simulink model "bh_compare_SM_vs_HAND_quad_and_spin_props"  (R2021b)
settings: Solver=ode23t  StartTime=0.0  StopTime=200  FixedStep=0.001  RelTol=1e-5  EnableMultiTasking=on
undefined symbols (not defined in the file or in its folder): P_elec, P_mot, P_one_prop, P_rot, P_veh, P_veh_no_props, sigbuilder_block, X, xme_dot_0, Y, Z
libraries: fl_lib x85, simulink_extras x40, nesl_utility x35, slpidlib x24, bh_6dof_LIBRARY x24, sm_lib x23, fl_ps_legacy_lib x7, simulink x2
(part 4 of 6)

== system bh_compare_SM_vs_HAND_quad_and_spin_props/CONT_SYS W_MOT_CMDS/MOTOR_sys/MOTOR_1 ==
  note: motor with PROPELLER
  w_CMD : Inport
  Bus Selector1 : BusSelector  OutputSignals=Elec.i,TQ_mot.Kt_i
  Lift : Scope  NumInputPorts=3
  MOTOR_PARAMS_STRUCT : bh_6dof_LIBRARY/MODELS/DC Motor_and_gearhead  K=P_mot.Ka  B=P_mot.b  J=P_mot.I  R=P_mot.R  L=P_mot.L  Kb=P_mot.Ke  ID=P_mot.ID
  Mux : Mux  Inputs=2
  PI_CONT : slpidlib/PID Controller  Controller=PI  Form=Parallel  TimeDomain=Continuous-time  UseExternalTs=off  SampleTime=-1  IntegratorMethod=Forward Euler  FilterMethod=Forward Euler  ControllerParametersSource=internal  P=2.97678216835849  I=24.9655384194189  D=-0.0417302954853434  UseFilter=on  N=6.67624174583517  TunerSelectOption=Transfer Function Based (PID Tuner App)  InitialConditionSource=internal  InitialConditionForIntegrator=0  InitialConditionForFilter=0  DifferentiatorICPrevScaledInput=0  ExternalReset=none  TrackingMode=off  Kt=1  LimitOutput=off  SatLimitsSource=internal  UpperSaturationLimit=inf  LowerSaturationLimit=-inf  LinearizeAsGain=on  AntiWindupMode=none  Kb=1  POutMin=[]  POutMax=[]  IOutMin=[]  IOutMax=[]  DOutMin=[]  DOutMax=[]  NOutMin=[]  NOutMax=[]  SumOutMin=[]  SumOutMax=[]  SaturationOutMin=[]  SaturationOutMax=[]  PParamMin=[]  PParamMax=[]  IParamMin=[]  IParamMax=[]  DParamMin=[]  DParamMax=[]  NParamMin=[]  NParamMax=[]  KbParamMin=[]  KbParamMax=[]  KtParamMin=[]  KtParamMax=[]  KbOutMin=[]  KbOutMax=[]  KtOutMin=[]  KtOutMax=[]  IntegratorOutMin=[]  IntegratorOutMax=[]  FilterOutMin=[]  FilterOutMax=[]  SumI1OutMin=[]  SumI1OutMax=[]  SumI2OutMin=[]  SumI2OutMax=[]  SumI3OutMin=[]  SumI3OutMax=[]  SumI4OutMin=[]  SumI4OutMax=[]  SumDOutMin=[]  SumDOutMax=[]  DifferentiatorOutMin=[]  DifferentiatorOutMax=[]  FilterDiffOutCoefMin=[]  FilterDiffOutCoefMax=[]  ReciprocalOutMin=[]  ReciprocalOutMax=[]  SumDenOutMin=[]  SumDenOutMax=[]  SumNumOutMin=[]  SumNumOutMax=[]  DivideOutMin=[]  DivideOutMax=[]  UdiffTsProdOutMin=[]  UdiffTsProdOutMax=[]  NTsProdOutMin=[]  NTsProdOutMax=[]  UintegralTsProdOutMin=[]  UintegralTsProdOutMax=[]  UngainTsProdOutMin=[]  UngainTsProdOutMax=[]  IntegratorContinuousStateAttributes=''  IntegratorStateMustResolveToSignalObject=off  IntegratorRTWStateStorageClass=Auto  FilterContinuousStateAttributes=''  FilterStateMustResolveToSignalObject=off  FilterRTWStateStorageClass=Auto  ParallelPVariant=InternalParameters  IdealPVariant=Disabled  IVariant=InternalParameters  DVariant=Disabled  IntegratorVariant=Continuous  SatVariant=Disabled  AWVariant=Passthrough  PCopyVariant=Disabled  TRVariant=Disabled  FdbkBlocksVariant=Forward  IdealPFdbkVariant=Disabled  SatFdbkVariant=Disabled  DerivativeFilterVariant=Disabled  NVariant=Disabled  NCopyVariant=Disabled_SignalSpec  FilterICVariant=Disabled  IntegratorICVariant=InternalICs  ExternalResetVariant=Disabled  TRSumVariant=Passthrough  SumFdbkVariant=Disabled  SumVariant=Sum_PI  TsampFilterVariant=InternalTs  TsampNgainVariant=Passthrough  TsampIntegralVariant=Passthrough  ExternalSaturationOutDataTypeStr=Inherit: Same as second input
  RPS_Lift_TG_drag : Scope  NumInputPorts=3
  Scope3 : Scope  NumInputPorts=4
  Sum1 : Sum  Inputs=|+-
  Terminator : Terminator
  VOLTAGE Saturation : Saturate  UpperLimit=P_elec.V_mot_max  LowerLimit=P_elec.V_mot_min
      settings: AttributesFormatString=|
      | Vmax = %<UpperLimit>
      | Vmin = %<LowerLimit>
  prefilter : Subsystem  mask(Derivative Estimation){wn=2*pi*5, p=1}
      mask prompts: wn "Natural frequency, wn (rad/sec)"; p "Damping ratio, p"
      mask help:
      | A simple derivative estimator using a 2nd order representation between input and output.
      |
      | The integrators use a discrete FORWARd Euler rule, and a sample time needs to be specified.
      mask init:
      | str1 = sprintf('wn = %.2f', wn);
      | str2 = sprintf('p  = %.2f', p);
      | %str3 = sprintf('dt = %.2f', dt);
      | %str = char(str1,str2,str3);
      | %str3 = sprintf('dt = %.2f', dt);
      | str = char(str1,str2);
      mask Display: disp(str)
  w_to_RPS : bh_6dof_LIBRARY/MODELS/w_to_RPS  SystemSampleTime=-1  VariantActivationTime=update diagram  Latency=0  AutoFrameSizeCalculation=off
  w_to_RPS1 : bh_6dof_LIBRARY/MODELS/w_to_RPS  SystemSampleTime=-1  VariantActivationTime=update diagram  Latency=0  AutoFrameSizeCalculation=off
  w_to_TQ_drag : bh_6dof_LIBRARY/MODELS/w_to_TQ_drag  k=P_one_prop.TWIST_per_w2
  w_to_Thrust : bh_6dof_LIBRARY/MODELS/w_to_Thrust  k=P_one_prop.LIFT_per_w2
  w : Outport  VectorParamsAs1DForOutWhenUnconnected=off
  wires:
  VOLTAGE Saturation/1 -> Lift/1, MOTOR_PARAMS_STRUCT/1  "VOLTS"
  [TQdrag] -> RPS_Lift_TG_drag/3  "TQdrag"
  Sum1/1 -> PI_CONT/1
  w_to_TQ_drag/1 -> [TQdrag], MOTOR_PARAMS_STRUCT/2, Scope3/4
  [LIFT] -> RPS_Lift_TG_drag/2  "LIFT"
  [wRPS_YES_prop] -> RPS_Lift_TG_drag/1  "RPS"
  w_to_Thrust/1 -> [LIFT]
  w_to_RPS/1 -> [wRPS_YES_prop], Scope3/1  "RPS"
  Bus Selector1/1 -> Scope3/2  "<i>"
  MOTOR_PARAMS_STRUCT/2 -> Bus Selector1/1
  Bus Selector1/2 -> Scope3/3  "<Kt_i>"
  MOTOR_PARAMS_STRUCT/1 -> w_to_RPS/1, [w], w/1, w_to_Thrust/1, w_to_TQ_drag/1
  [w] -> Sum1/2
  [LIFT] -> Lift/2  "LIFT"
  Mux/1 -> w_to_RPS1/1  "w"
  [w] -> Mux/2
  w_to_RPS1/1 -> Lift/3  "w_RPS"
  PI_CONT/1 -> VOLTAGE Saturation/1  "VOLTS"
  w_CMD/1 -> prefilter/1(U)  "w_rad_per_sec"
  prefilter/1(U_filt) -> Mux/1, Sum1/1
  prefilter/2(U_DOT) -> Terminator/1

== system bh_compare_SM_vs_HAND_quad_and_spin_props/CONT_SYS W_MOT_CMDS/MOTOR_sys/MOTOR_2 ==
  note: motor with PROPELLER
  w_CMD : Inport
  Bus Selector1 : BusSelector  OutputSignals=Elec.i,TQ_mot.Kt_i
  Lift : Scope  NumInputPorts=3
  MOTOR_PARAMS_STRUCT : bh_6dof_LIBRARY/MODELS/DC Motor_and_gearhead  K=P_mot.Ka  B=P_mot.b  J=P_mot.I  R=P_mot.R  L=P_mot.L  Kb=P_mot.Ke  ID=P_mot.ID
  Mux : Mux  Inputs=2
  PI_CONT : slpidlib/PID Controller  Controller=PI  Form=Parallel  TimeDomain=Continuous-time  UseExternalTs=off  SampleTime=-1  IntegratorMethod=Forward Euler  FilterMethod=Forward Euler  ControllerParametersSource=internal  P=2.97678216835849  I=24.9655384194189  D=-0.0417302954853434  UseFilter=on  N=6.67624174583517  TunerSelectOption=Transfer Function Based (PID Tuner App)  InitialConditionSource=internal  InitialConditionForIntegrator=0  InitialConditionForFilter=0  DifferentiatorICPrevScaledInput=0  ExternalReset=none  TrackingMode=off  Kt=1  LimitOutput=off  SatLimitsSource=internal  UpperSaturationLimit=inf  LowerSaturationLimit=-inf  LinearizeAsGain=on  AntiWindupMode=none  Kb=1  POutMin=[]  POutMax=[]  IOutMin=[]  IOutMax=[]  DOutMin=[]  DOutMax=[]  NOutMin=[]  NOutMax=[]  SumOutMin=[]  SumOutMax=[]  SaturationOutMin=[]  SaturationOutMax=[]  PParamMin=[]  PParamMax=[]  IParamMin=[]  IParamMax=[]  DParamMin=[]  DParamMax=[]  NParamMin=[]  NParamMax=[]  KbParamMin=[]  KbParamMax=[]  KtParamMin=[]  KtParamMax=[]  KbOutMin=[]  KbOutMax=[]  KtOutMin=[]  KtOutMax=[]  IntegratorOutMin=[]  IntegratorOutMax=[]  FilterOutMin=[]  FilterOutMax=[]  SumI1OutMin=[]  SumI1OutMax=[]  SumI2OutMin=[]  SumI2OutMax=[]  SumI3OutMin=[]  SumI3OutMax=[]  SumI4OutMin=[]  SumI4OutMax=[]  SumDOutMin=[]  SumDOutMax=[]  DifferentiatorOutMin=[]  DifferentiatorOutMax=[]  FilterDiffOutCoefMin=[]  FilterDiffOutCoefMax=[]  ReciprocalOutMin=[]  ReciprocalOutMax=[]  SumDenOutMin=[]  SumDenOutMax=[]  SumNumOutMin=[]  SumNumOutMax=[]  DivideOutMin=[]  DivideOutMax=[]  UdiffTsProdOutMin=[]  UdiffTsProdOutMax=[]  NTsProdOutMin=[]  NTsProdOutMax=[]  UintegralTsProdOutMin=[]  UintegralTsProdOutMax=[]  UngainTsProdOutMin=[]  UngainTsProdOutMax=[]  IntegratorContinuousStateAttributes=''  IntegratorStateMustResolveToSignalObject=off  IntegratorRTWStateStorageClass=Auto  FilterContinuousStateAttributes=''  FilterStateMustResolveToSignalObject=off  FilterRTWStateStorageClass=Auto  ParallelPVariant=InternalParameters  IdealPVariant=Disabled  IVariant=InternalParameters  DVariant=Disabled  IntegratorVariant=Continuous  SatVariant=Disabled  AWVariant=Passthrough  PCopyVariant=Disabled  TRVariant=Disabled  FdbkBlocksVariant=Forward  IdealPFdbkVariant=Disabled  SatFdbkVariant=Disabled  DerivativeFilterVariant=Disabled  NVariant=Disabled  NCopyVariant=Disabled_SignalSpec  FilterICVariant=Disabled  IntegratorICVariant=InternalICs  ExternalResetVariant=Disabled  TRSumVariant=Passthrough  SumFdbkVariant=Disabled  SumVariant=Sum_PI  TsampFilterVariant=InternalTs  TsampNgainVariant=Passthrough  TsampIntegralVariant=Passthrough  ExternalSaturationOutDataTypeStr=Inherit: Same as second input
  RPS_Lift_TG_drag : Scope  NumInputPorts=3
  Scope3 : Scope  NumInputPorts=4
  Sum1 : Sum  Inputs=|+-
  Terminator : Terminator
  VOLTAGE Saturation : Saturate  UpperLimit=P_elec.V_mot_max  LowerLimit=P_elec.V_mot_min
      settings: AttributesFormatString=|
      | Vmax = %<UpperLimit>
      | Vmin = %<LowerLimit>
  prefilter : Subsystem  mask(Derivative Estimation){wn=2*pi*5, p=1}
      mask prompts: wn "Natural frequency, wn (rad/sec)"; p "Damping ratio, p"
      mask help:
      | A simple derivative estimator using a 2nd order representation between input and output.
      |
      | The integrators use a discrete FORWARd Euler rule, and a sample time needs to be specified.
      mask init:
      | str1 = sprintf('wn = %.2f', wn);
      | str2 = sprintf('p  = %.2f', p);
      | %str3 = sprintf('dt = %.2f', dt);
      | %str = char(str1,str2,str3);
      | %str3 = sprintf('dt = %.2f', dt);
      | str = char(str1,str2);
      mask Display: disp(str)
  w_to_RPS : bh_6dof_LIBRARY/MODELS/w_to_RPS  SystemSampleTime=-1  VariantActivationTime=update diagram  Latency=0  AutoFrameSizeCalculation=off
  w_to_RPS1 : bh_6dof_LIBRARY/MODELS/w_to_RPS  SystemSampleTime=-1  VariantActivationTime=update diagram  Latency=0  AutoFrameSizeCalculation=off
  w_to_TQ_drag : bh_6dof_LIBRARY/MODELS/w_to_TQ_drag  k=P_one_prop.TWIST_per_w2
  w_to_Thrust : bh_6dof_LIBRARY/MODELS/w_to_Thrust  k=P_one_prop.LIFT_per_w2
  w : Outport  VectorParamsAs1DForOutWhenUnconnected=off
  wires:
  VOLTAGE Saturation/1 -> Lift/1, MOTOR_PARAMS_STRUCT/1  "VOLTS"
  [TQdrag] -> RPS_Lift_TG_drag/3  "TQdrag"
  Sum1/1 -> PI_CONT/1
  w_to_TQ_drag/1 -> [TQdrag], MOTOR_PARAMS_STRUCT/2, Scope3/4
  [LIFT] -> RPS_Lift_TG_drag/2  "LIFT"
  [wRPS_YES_prop] -> RPS_Lift_TG_drag/1  "RPS"
  w_to_Thrust/1 -> [LIFT]
  w_to_RPS/1 -> [wRPS_YES_prop], Scope3/1  "RPS"
  Bus Selector1/1 -> Scope3/2  "<i>"
  MOTOR_PARAMS_STRUCT/2 -> Bus Selector1/1
  Bus Selector1/2 -> Scope3/3  "<Kt_i>"
  MOTOR_PARAMS_STRUCT/1 -> w_to_RPS/1, [w], w/1, w_to_Thrust/1, w_to_TQ_drag/1
  [w] -> Sum1/2
  [LIFT] -> Lift/2  "LIFT"
  Mux/1 -> w_to_RPS1/1  "w"
  [w] -> Mux/2
  w_to_RPS1/1 -> Lift/3  "w_RPS"
  PI_CONT/1 -> VOLTAGE Saturation/1  "VOLTS"
  w_CMD/1 -> prefilter/1(U)  "w_rad_per_sec"
  prefilter/1(U_filt) -> Mux/1, Sum1/1
  prefilter/2(U_DOT) -> Terminator/1

== system bh_compare_SM_vs_HAND_quad_and_spin_props/CONT_SYS W_MOT_CMDS/MOTOR_sys/MOTOR_3 ==
  note: motor with PROPELLER
  w_CMD : Inport
  Bus Selector1 : BusSelector  OutputSignals=Elec.i,TQ_mot.Kt_i
  Lift : Scope  NumInputPorts=3
  MOTOR_PARAMS_STRUCT : bh_6dof_LIBRARY/MODELS/DC Motor_and_gearhead  K=P_mot.Ka  B=P_mot.b  J=P_mot.I  R=P_mot.R  L=P_mot.L  Kb=P_mot.Ke  ID=P_mot.ID
  Mux : Mux  Inputs=2
  PI_CONT : slpidlib/PID Controller  Controller=PI  Form=Parallel  TimeDomain=Continuous-time  UseExternalTs=off  SampleTime=-1  IntegratorMethod=Forward Euler  FilterMethod=Forward Euler  ControllerParametersSource=internal  P=2.97678216835849  I=24.9655384194189  D=-0.0417302954853434  UseFilter=on  N=6.67624174583517  TunerSelectOption=Transfer Function Based (PID Tuner App)  InitialConditionSource=internal  InitialConditionForIntegrator=0  InitialConditionForFilter=0  DifferentiatorICPrevScaledInput=0  ExternalReset=none  TrackingMode=off  Kt=1  LimitOutput=off  SatLimitsSource=internal  UpperSaturationLimit=inf  LowerSaturationLimit=-inf  LinearizeAsGain=on  AntiWindupMode=none  Kb=1  POutMin=[]  POutMax=[]  IOutMin=[]  IOutMax=[]  DOutMin=[]  DOutMax=[]  NOutMin=[]  NOutMax=[]  SumOutMin=[]  SumOutMax=[]  SaturationOutMin=[]  SaturationOutMax=[]  PParamMin=[]  PParamMax=[]  IParamMin=[]  IParamMax=[]  DParamMin=[]  DParamMax=[]  NParamMin=[]  NParamMax=[]  KbParamMin=[]  KbParamMax=[]  KtParamMin=[]  KtParamMax=[]  KbOutMin=[]  KbOutMax=[]  KtOutMin=[]  KtOutMax=[]  IntegratorOutMin=[]  IntegratorOutMax=[]  FilterOutMin=[]  FilterOutMax=[]  SumI1OutMin=[]  SumI1OutMax=[]  SumI2OutMin=[]  SumI2OutMax=[]  SumI3OutMin=[]  SumI3OutMax=[]  SumI4OutMin=[]  SumI4OutMax=[]  SumDOutMin=[]  SumDOutMax=[]  DifferentiatorOutMin=[]  DifferentiatorOutMax=[]  FilterDiffOutCoefMin=[]  FilterDiffOutCoefMax=[]  ReciprocalOutMin=[]  ReciprocalOutMax=[]  SumDenOutMin=[]  SumDenOutMax=[]  SumNumOutMin=[]  SumNumOutMax=[]  DivideOutMin=[]  DivideOutMax=[]  UdiffTsProdOutMin=[]  UdiffTsProdOutMax=[]  NTsProdOutMin=[]  NTsProdOutMax=[]  UintegralTsProdOutMin=[]  UintegralTsProdOutMax=[]  UngainTsProdOutMin=[]  UngainTsProdOutMax=[]  IntegratorContinuousStateAttributes=''  IntegratorStateMustResolveToSignalObject=off  IntegratorRTWStateStorageClass=Auto  FilterContinuousStateAttributes=''  FilterStateMustResolveToSignalObject=off  FilterRTWStateStorageClass=Auto  ParallelPVariant=InternalParameters  IdealPVariant=Disabled  IVariant=InternalParameters  DVariant=Disabled  IntegratorVariant=Continuous  SatVariant=Disabled  AWVariant=Passthrough  PCopyVariant=Disabled  TRVariant=Disabled  FdbkBlocksVariant=Forward  IdealPFdbkVariant=Disabled  SatFdbkVariant=Disabled  DerivativeFilterVariant=Disabled  NVariant=Disabled  NCopyVariant=Disabled_SignalSpec  FilterICVariant=Disabled  IntegratorICVariant=InternalICs  ExternalResetVariant=Disabled  TRSumVariant=Passthrough  SumFdbkVariant=Disabled  SumVariant=Sum_PI  TsampFilterVariant=InternalTs  TsampNgainVariant=Passthrough  TsampIntegralVariant=Passthrough  ExternalSaturationOutDataTypeStr=Inherit: Same as second input
  RPS_Lift_TG_drag : Scope  NumInputPorts=3
  Scope3 : Scope  NumInputPorts=4
  Sum1 : Sum  Inputs=|+-
  Terminator : Terminator
  VOLTAGE Saturation : Saturate  UpperLimit=P_elec.V_mot_max  LowerLimit=P_elec.V_mot_min
      settings: AttributesFormatString=|
      | Vmax = %<UpperLimit>
      | Vmin = %<LowerLimit>
  prefilter : Subsystem  mask(Derivative Estimation){wn=2*pi*5, p=1}
      mask prompts: wn "Natural frequency, wn (rad/sec)"; p "Damping ratio, p"
      mask help:
      | A simple derivative estimator using a 2nd order representation between input and output.
      |
      | The integrators use a discrete FORWARd Euler rule, and a sample time needs to be specified.
      mask init:
      | str1 = sprintf('wn = %.2f', wn);
      | str2 = sprintf('p  = %.2f', p);
      | %str3 = sprintf('dt = %.2f', dt);
      | %str = char(str1,str2,str3);
      | %str3 = sprintf('dt = %.2f', dt);
      | str = char(str1,str2);
      mask Display: disp(str)
  w_to_RPS : bh_6dof_LIBRARY/MODELS/w_to_RPS  SystemSampleTime=-1  VariantActivationTime=update diagram  Latency=0  AutoFrameSizeCalculation=off
  w_to_RPS1 : bh_6dof_LIBRARY/MODELS/w_to_RPS  SystemSampleTime=-1  VariantActivationTime=update diagram  Latency=0  AutoFrameSizeCalculation=off
  w_to_TQ_drag : bh_6dof_LIBRARY/MODELS/w_to_TQ_drag  k=P_one_prop.TWIST_per_w2
  w_to_Thrust : bh_6dof_LIBRARY/MODELS/w_to_Thrust  k=P_one_prop.LIFT_per_w2
  w : Outport  VectorParamsAs1DForOutWhenUnconnected=off
  wires:
  VOLTAGE Saturation/1 -> Lift/1, MOTOR_PARAMS_STRUCT/1  "VOLTS"
  [TQdrag] -> RPS_Lift_TG_drag/3  "TQdrag"
  Sum1/1 -> PI_CONT/1
  w_to_TQ_drag/1 -> [TQdrag], MOTOR_PARAMS_STRUCT/2, Scope3/4
  [LIFT] -> RPS_Lift_TG_drag/2  "LIFT"
  [wRPS_YES_prop] -> RPS_Lift_TG_drag/1  "RPS"
  w_to_Thrust/1 -> [LIFT]
  w_to_RPS/1 -> [wRPS_YES_prop], Scope3/1  "RPS"
  Bus Selector1/1 -> Scope3/2  "<i>"
  MOTOR_PARAMS_STRUCT/2 -> Bus Selector1/1
  Bus Selector1/2 -> Scope3/3  "<Kt_i>"
  MOTOR_PARAMS_STRUCT/1 -> w_to_RPS/1, [w], w/1, w_to_Thrust/1, w_to_TQ_drag/1
  [w] -> Sum1/2
  [LIFT] -> Lift/2  "LIFT"
  Mux/1 -> w_to_RPS1/1  "w"
  [w] -> Mux/2
  w_to_RPS1/1 -> Lift/3  "w_RPS"
  PI_CONT/1 -> VOLTAGE Saturation/1  "VOLTS"
  w_CMD/1 -> prefilter/1(U)  "w_rad_per_sec"
  prefilter/1(U_filt) -> Mux/1, Sum1/1
  prefilter/2(U_DOT) -> Terminator/1

== system bh_compare_SM_vs_HAND_quad_and_spin_props/CONT_SYS W_MOT_CMDS/MOTOR_sys/MOTOR_4 ==
  note: motor with PROPELLER
  w_CMD : Inport
  Bus Selector1 : BusSelector  OutputSignals=Elec.i,TQ_mot.Kt_i
  Lift : Scope  NumInputPorts=3
  MOTOR_PARAMS_STRUCT : bh_6dof_LIBRARY/MODELS/DC Motor_and_gearhead  K=P_mot.Ka  B=P_mot.b  J=P_mot.I  R=P_mot.R  L=P_mot.L  Kb=P_mot.Ke  ID=P_mot.ID
  Mux : Mux  Inputs=2
  PI_CONT : slpidlib/PID Controller  Controller=PI  Form=Parallel  TimeDomain=Continuous-time  UseExternalTs=off  SampleTime=-1  IntegratorMethod=Forward Euler  FilterMethod=Forward Euler  ControllerParametersSource=internal  P=2.97678216835849  I=24.9655384194189  D=-0.0417302954853434  UseFilter=on  N=6.67624174583517  TunerSelectOption=Transfer Function Based (PID Tuner App)  InitialConditionSource=internal  InitialConditionForIntegrator=0  InitialConditionForFilter=0  DifferentiatorICPrevScaledInput=0  ExternalReset=none  TrackingMode=off  Kt=1  LimitOutput=off  SatLimitsSource=internal  UpperSaturationLimit=inf  LowerSaturationLimit=-inf  LinearizeAsGain=on  AntiWindupMode=none  Kb=1  POutMin=[]  POutMax=[]  IOutMin=[]  IOutMax=[]  DOutMin=[]  DOutMax=[]  NOutMin=[]  NOutMax=[]  SumOutMin=[]  SumOutMax=[]  SaturationOutMin=[]  SaturationOutMax=[]  PParamMin=[]  PParamMax=[]  IParamMin=[]  IParamMax=[]  DParamMin=[]  DParamMax=[]  NParamMin=[]  NParamMax=[]  KbParamMin=[]  KbParamMax=[]  KtParamMin=[]  KtParamMax=[]  KbOutMin=[]  KbOutMax=[]  KtOutMin=[]  KtOutMax=[]  IntegratorOutMin=[]  IntegratorOutMax=[]  FilterOutMin=[]  FilterOutMax=[]  SumI1OutMin=[]  SumI1OutMax=[]  SumI2OutMin=[]  SumI2OutMax=[]  SumI3OutMin=[]  SumI3OutMax=[]  SumI4OutMin=[]  SumI4OutMax=[]  SumDOutMin=[]  SumDOutMax=[]  DifferentiatorOutMin=[]  DifferentiatorOutMax=[]  FilterDiffOutCoefMin=[]  FilterDiffOutCoefMax=[]  ReciprocalOutMin=[]  ReciprocalOutMax=[]  SumDenOutMin=[]  SumDenOutMax=[]  SumNumOutMin=[]  SumNumOutMax=[]  DivideOutMin=[]  DivideOutMax=[]  UdiffTsProdOutMin=[]  UdiffTsProdOutMax=[]  NTsProdOutMin=[]  NTsProdOutMax=[]  UintegralTsProdOutMin=[]  UintegralTsProdOutMax=[]  UngainTsProdOutMin=[]  UngainTsProdOutMax=[]  IntegratorContinuousStateAttributes=''  IntegratorStateMustResolveToSignalObject=off  IntegratorRTWStateStorageClass=Auto  FilterContinuousStateAttributes=''  FilterStateMustResolveToSignalObject=off  FilterRTWStateStorageClass=Auto  ParallelPVariant=InternalParameters  IdealPVariant=Disabled  IVariant=InternalParameters  DVariant=Disabled  IntegratorVariant=Continuous  SatVariant=Disabled  AWVariant=Passthrough  PCopyVariant=Disabled  TRVariant=Disabled  FdbkBlocksVariant=Forward  IdealPFdbkVariant=Disabled  SatFdbkVariant=Disabled  DerivativeFilterVariant=Disabled  NVariant=Disabled  NCopyVariant=Disabled_SignalSpec  FilterICVariant=Disabled  IntegratorICVariant=InternalICs  ExternalResetVariant=Disabled  TRSumVariant=Passthrough  SumFdbkVariant=Disabled  SumVariant=Sum_PI  TsampFilterVariant=InternalTs  TsampNgainVariant=Passthrough  TsampIntegralVariant=Passthrough  ExternalSaturationOutDataTypeStr=Inherit: Same as second input
  RPS_Lift_TG_drag : Scope  NumInputPorts=3
  Scope3 : Scope  NumInputPorts=4
  Sum1 : Sum  Inputs=|+-
  Terminator : Terminator
  VOLTAGE Saturation : Saturate  UpperLimit=P_elec.V_mot_max  LowerLimit=P_elec.V_mot_min
      settings: AttributesFormatString=|
      | Vmax = %<UpperLimit>
      | Vmin = %<LowerLimit>
  prefilter : Subsystem  mask(Derivative Estimation){wn=2*pi*5, p=1}
      mask prompts: wn "Natural frequency, wn (rad/sec)"; p "Damping ratio, p"
      mask help:
      | A simple derivative estimator using a 2nd order representation between input and output.
      |
      | The integrators use a discrete FORWARd Euler rule, and a sample time needs to be specified.
      mask init:
      | str1 = sprintf('wn = %.2f', wn);
      | str2 = sprintf('p  = %.2f', p);
      | %str3 = sprintf('dt = %.2f', dt);
      | %str = char(str1,str2,str3);
      | %str3 = sprintf('dt = %.2f', dt);
      | str = char(str1,str2);
      mask Display: disp(str)
  w_to_RPS : bh_6dof_LIBRARY/MODELS/w_to_RPS  SystemSampleTime=-1  VariantActivationTime=update diagram  Latency=0  AutoFrameSizeCalculation=off
  w_to_RPS1 : bh_6dof_LIBRARY/MODELS/w_to_RPS  SystemSampleTime=-1  VariantActivationTime=update diagram  Latency=0  AutoFrameSizeCalculation=off
  w_to_TQ_drag : bh_6dof_LIBRARY/MODELS/w_to_TQ_drag  k=P_one_prop.TWIST_per_w2
  w_to_Thrust : bh_6dof_LIBRARY/MODELS/w_to_Thrust  k=P_one_prop.LIFT_per_w2
  w : Outport  VectorParamsAs1DForOutWhenUnconnected=off
  wires:
  VOLTAGE Saturation/1 -> Lift/1, MOTOR_PARAMS_STRUCT/1  "VOLTS"
  [TQdrag] -> RPS_Lift_TG_drag/3  "TQdrag"
  Sum1/1 -> PI_CONT/1
  w_to_TQ_drag/1 -> [TQdrag], MOTOR_PARAMS_STRUCT/2, Scope3/4
  [LIFT] -> RPS_Lift_TG_drag/2  "LIFT"
  [wRPS_YES_prop] -> RPS_Lift_TG_drag/1  "RPS"
  w_to_Thrust/1 -> [LIFT]
  w_to_RPS/1 -> [wRPS_YES_prop], Scope3/1  "RPS"
  Bus Selector1/1 -> Scope3/2  "<i>"
  MOTOR_PARAMS_STRUCT/2 -> Bus Selector1/1
  Bus Selector1/2 -> Scope3/3  "<Kt_i>"
  MOTOR_PARAMS_STRUCT/1 -> w_to_RPS/1, [w], w/1, w_to_Thrust/1, w_to_TQ_drag/1
  [w] -> Sum1/2
  [LIFT] -> Lift/2  "LIFT"
  Mux/1 -> w_to_RPS1/1  "w"
  [w] -> Mux/2
  w_to_RPS1/1 -> Lift/3  "w_RPS"
  PI_CONT/1 -> VOLTAGE Saturation/1  "VOLTS"
  w_CMD/1 -> prefilter/1(U)  "w_rad_per_sec"
  prefilter/1(U_filt) -> Mux/1, Sum1/1
  prefilter/2(U_DOT) -> Terminator/1

== system bh_compare_SM_vs_HAND_quad_and_spin_props/CONT_SYS W_MOT_CMDS/MOTOR_sys/w_MUX ==
  W_CMD : Inport
  W : Inport  Port=2
  Demux1 : Demux
  Demux2 : Demux
  Mux{,1..3} (4 alike) : Mux  Inputs=2
  w1 : Outport  VectorParamsAs1DForOutWhenUnconnected=off
  w2 : Outport  Port=2  VectorParamsAs1DForOutWhenUnconnected=off
  w3 : Outport  Port=3  VectorParamsAs1DForOutWhenUnconnected=off
  w4 : Outport  Port=4  VectorParamsAs1DForOutWhenUnconnected=off
  wires:
  W_CMD/1 -> Demux2/1
  W/1 -> Demux1/1
  Mux/1 -> w1/1
  Mux1/1 -> w2/1
  Mux3/1 -> w4/1
  Mux2/1 -> w3/1
  Demux2/1 -> Mux/1
  Demux2/2 -> Mux1/1
  Demux2/3 -> Mux2/1
  Demux2/4 -> Mux3/1
  Demux1/1 -> Mux/2
  Demux1/2 -> Mux1/2
  Demux1/3 -> Mux2/2
  Demux1/4 -> Mux3/2

== system bh_compare_SM_vs_HAND_quad_and_spin_props/CONT_SYS W_MOT_CMDS2/PRE_FILTERS/prefilter ==
  note: Y = U *     wn^2/( s^2 + 2*p*wn*s + wn^2)
      | Y*( s^2 + 2*p*wn*s + wn^2) = U * wn^2
      |
      | y'' + y'*2*p*wn + y*wn^2 = U*wn^2
  U : Inport
  Gain : Gain  Gain=2*p*wn
  Gain1 : Gain  Gain=wn^2
  Gain2 : Gain  Gain=wn^2
  Integrator : Integrator
  Integrator1 : Integrator
  Sum : Sum  Inputs=|+--
  U_filt : Outport  VectorParamsAs1DForOutWhenUnconnected=off
  U_DOT : Outport  Port=2  VectorParamsAs1DForOutWhenUnconnected=off
  wires:
  Integrator/1 -> Integrator1/1, [Y_DOT], Gain/1  "y_dot"
  Sum/1 -> Integrator/1  "y_dot_dot"
  Integrator1/1 -> Gain1/1, U_filt/1  "y"
  U/1 -> Gain2/1
  Gain2/1 -> Sum/1
  Gain/1 -> Sum/3
  Gain1/1 -> Sum/2
  [Y_DOT] -> U_DOT/1

== system bh_compare_SM_vs_HAND_quad_and_spin_props/CONT_SYS W_MOT_CMDS2/PRE_FILTERS/prefilter1 ==
  note: Y = U *     wn^2/( s^2 + 2*p*wn*s + wn^2)
      | Y*( s^2 + 2*p*wn*s + wn^2) = U * wn^2
      |
      | y'' + y'*2*p*wn + y*wn^2 = U*wn^2
  U : Inport
  Gain : Gain  Gain=2*p*wn
  Gain1 : Gain  Gain=wn^2
  Gain2 : Gain  Gain=wn^2
  Integrator : Integrator
  Integrator1 : Integrator
  Sum : Sum  Inputs=|+--
  U_filt : Outport  VectorParamsAs1DForOutWhenUnconnected=off
  U_DOT : Outport  Port=2  VectorParamsAs1DForOutWhenUnconnected=off
  wires:
  Integrator/1 -> Integrator1/1, [Y_DOT], Gain/1  "y_dot"
  Sum/1 -> Integrator/1  "y_dot_dot"
  Integrator1/1 -> Gain1/1, U_filt/1  "y"
  U/1 -> Gain2/1
  Gain2/1 -> Sum/1
  Gain/1 -> Sum/3
  Gain1/1 -> Sum/2
  [Y_DOT] -> U_DOT/1

== system bh_compare_SM_vs_HAND_quad_and_spin_props/CONT_SYS W_MOT_CMDS2/PRE_FILTERS/prefilter2 ==
  note: Y = U *     wn^2/( s^2 + 2*p*wn*s + wn^2)
      | Y*( s^2 + 2*p*wn*s + wn^2) = U * wn^2
      |
      | y'' + y'*2*p*wn + y*wn^2 = U*wn^2
  U : Inport
  Gain : Gain  Gain=2*p*wn
  Gain1 : Gain  Gain=wn^2
  Gain2 : Gain  Gain=wn^2
  Integrator : Integrator
  Integrator1 : Integrator
  Sum : Sum  Inputs=|+--
  U_filt : Outport  VectorParamsAs1DForOutWhenUnconnected=off
  U_DOT : Outport  Port=2  VectorParamsAs1DForOutWhenUnconnected=off
  wires:
  Integrator/1 -> Integrator1/1, [Y_DOT], Gain/1  "y_dot"
  Sum/1 -> Integrator/1  "y_dot_dot"
  Integrator1/1 -> Gain1/1, U_filt/1  "y"
  U/1 -> Gain2/1
  Gain2/1 -> Sum/1
  Gain/1 -> Sum/3
  Gain1/1 -> Sum/2
  [Y_DOT] -> U_DOT/1

== system bh_compare_SM_vs_HAND_quad_and_spin_props/CONT_SYS W_MOT_CMDS2/PRE_FILTERS/prefilter3 ==
  note: Y = U *     wn^2/( s^2 + 2*p*wn*s + wn^2)
      | Y*( s^2 + 2*p*wn*s + wn^2) = U * wn^2
      |
      | y'' + y'*2*p*wn + y*wn^2 = U*wn^2
  U : Inport
  Gain : Gain  Gain=2*p*wn
  Gain1 : Gain  Gain=wn^2
  Gain2 : Gain  Gain=wn^2
  Integrator : Integrator
  Integrator1 : Integrator
  Sum : Sum  Inputs=|+--
  U_filt : Outport  VectorParamsAs1DForOutWhenUnconnected=off
  U_DOT : Outport  Port=2  VectorParamsAs1DForOutWhenUnconnected=off
  wires:
  Integrator/1 -> Integrator1/1, [Y_DOT], Gain/1  "y_dot"
  Sum/1 -> Integrator/1  "y_dot_dot"
  Integrator1/1 -> Gain1/1, U_filt/1  "y"
  U/1 -> Gain2/1
  Gain2/1 -> Sum/1
  Gain/1 -> Sum/3
  Gain1/1 -> Sum/2
  [Y_DOT] -> U_DOT/1

== system bh_compare_SM_vs_HAND_quad_and_spin_props/CONT_SYS W_MOT_CMDS2/PRE_FILTERS/w_MUX ==
  W_CMD : Inport
  W : Inport  Port=2
  Demux1 : Demux
  Demux2 : Demux
  Mux{,1..3} (4 alike) : Mux  Inputs=2
  w1 : Outport  VectorParamsAs1DForOutWhenUnconnected=off
  w2 : Outport  Port=2  VectorParamsAs1DForOutWhenUnconnected=off
  w3 : Outport  Port=3  VectorParamsAs1DForOutWhenUnconnected=off
  w4 : Outport  Port=4  VectorParamsAs1DForOutWhenUnconnected=off
  wires:
  W_CMD/1 -> Demux2/1
  W/1 -> Demux1/1
  Mux/1 -> w1/1
  Mux1/1 -> w2/1
  Mux3/1 -> w4/1
  Mux2/1 -> w3/1
  Demux2/1 -> Mux/1
  Demux2/2 -> Mux1/1
  Demux2/3 -> Mux2/1
  Demux2/4 -> Mux3/1
  Demux1/1 -> Mux/2
  Demux1/2 -> Mux1/2
  Demux1/3 -> Mux2/2
  Demux1/4 -> Mux3/2

== system bh_compare_SM_vs_HAND_quad_and_spin_props/MODEL_SYS/bh_6DOF (Simscape)/6DOF_JOINT_SYS ==
  note: NOTE:  For the 6-DOF block
      | SENSED positions and velocities are resolved into BASE frame components
      | INITIAL(target) positions and velocities are resolved into BASE frame components
  6-DOF Joint : sm_lib/Joints/6-DOF Joint  JointMode=Normal  SenseConstraintForce=off  SenseConstraintForceX=off  SenseConstraintForceY=off  SenseConstraintForceZ=off  SenseConstraintTorque=off  SenseConstraintTorqueX=off  SenseConstraintTorqueY=off  SenseConstraintTorqueZ=off  SenseTotalForce=off  SenseTotalForceX=off  SenseTotalForceY=off  SenseTotalForceZ=off  SenseTotalTorque=off  SenseTotalTorqueX=off  SenseTotalTorqueY=off  SenseTotalTorqueZ=off  CompositeWrenchDir=FollowerOnBase  CompositeWrenchFrame=BaseFrame  PxEquilibriumPosition=0  PxEquilibriumPositionUnits=m  PxSpringStiffness=0  PxSpringStiffnessUnits=N/m  PxDampingCoefficient=0  PxDampingCoefficientUnits=N/(m/s)  PxTorqueActuationMode=NoTorque  PxMotionActuationMode=ComputedMotion  PxSensePosition=on  PxSenseVelocity=on  PxSenseAcceleration=off  PxSenseTorqueForce=off  PxSenseLowerLimitTorqueForce=off  PxSenseUpperLimitTorqueForce=off  PxLowerLimitSpecify=off  PxLowerLimitBound=-1  PxLowerLimitBoundUnits=m  PxLowerLimitStiffness=1e6  PxLowerLimitStiffnessUnits=N/m  PxLowerLimitDamping=1e3  PxLowerLimitDampingUnits=N/(m/s)  PxLowerLimitTransitionRegionWidth=1e-4  PxLowerLimitTransitionRegionWidthUnits=m  PxUpperLimitSpecify=off  PxUpperLimitBound=1  PxUpperLimitBoundUnits=m  PxUpperLimitStiffness=1e6  PxUpperLimitStiffnessUnits=N/m  PxUpperLimitDamping=1e3  PxUpperLimitDampingUnits=N/(m/s)  PxUpperLimitTransitionRegionWidth=1e-4  PxUpperLimitTransitionRegionWidthUnits=m  PxPositionTargetSpecify=on  PxPositionTargetPriority=High  PxPositionTargetValue=xme_0(1)  PxPositionTargetValueUnits=m  PxVelocityTargetSpecify=on  PxVelocityTargetPriority=High  PxVelocityTargetValue=xme_dot_0(1)  PxVelocityTargetValueUnits=m/s  PyEquilibriumPosition=0  PyEquilibriumPositionUnits=m  PySpringStiffness=0  PySpringStiffnessUnits=N/m  PyDampingCoefficient=0  PyDampingCoefficientUnits=N/(m/s)  PyTorqueActuationMode=NoTorque  PyMotionActuationMode=ComputedMotion  PySensePosition=on  PySenseVelocity=on  PySenseAcceleration=off  PySenseTorqueForce=off  PySenseLowerLimitTorqueForce=off  PySenseUpperLimitTorqueForce=off  PyLowerLimitSpecify=off  PyLowerLimitBound=-1  PyLowerLimitBoundUnits=m  PyLowerLimitStiffness=1e6  PyLowerLimitStiffnessUnits=N/m  PyLowerLimitDamping=1e3  PyLowerLimitDampingUnits=N/(m/s)  PyLowerLimitTransitionRegionWidth=1e-4  PyLowerLimitTransitionRegionWidthUnits=m  PyUpperLimitSpecify=off  PyUpperLimitBound=1  PyUpperLimitBoundUnits=m  PyUpperLimitStiffness=1e6  PyUpperLimitStiffnessUnits=N/m  PyUpperLimitDamping=1e3  PyUpperLimitDampingUnits=N/(m/s)  PyUpperLimitTransitionRegionWidth=1e-4  PyUpperLimitTransitionRegionWidthUnits=m  PyPositionTargetSpecify=on  PyPositionTargetPriority=High  PyPositionTargetValue=xme_0(2)  PyPositionTargetValueUnits=m  PyVelocityTargetSpecify=on  PyVelocityTargetPriority=High  PyVelocityTargetValue=xme_dot_0(2)  PyVelocityTargetValueUnits=m/s  PzEquilibriumPosition=0  PzEquilibriumPositionUnits=m  PzSpringStiffness=0  PzSpringStiffnessUnits=N/m  PzDampingCoefficient=0  PzDampingCoefficientUnits=N/(m/s)  PzTorqueActuationMode=NoTorque  PzMotionActuationMode=ComputedMotion  PzSensePosition=on  PzSenseVelocity=on  PzSenseAcceleration=off  PzSenseTorqueForce=off  PzSenseLowerLimitTorqueForce=off  PzSenseUpperLimitTorqueForce=off  PzLowerLimitSpecify=off  PzLowerLimitBound=-1  PzLowerLimitBoundUnits=m  PzLowerLimitStiffness=1e6  PzLowerLimitStiffnessUnits=N/m  PzLowerLimitDamping=1e3  PzLowerLimitDampingUnits=N/(m/s)  PzLowerLimitTransitionRegionWidth=1e-4  PzLowerLimitTransitionRegionWidthUnits=m  PzUpperLimitSpecify=off  PzUpperLimitBound=1  PzUpperLimitBoundUnits=m  PzUpperLimitStiffness=1e6  PzUpperLimitStiffnessUnits=N/m  PzUpperLimitDamping=1e3  PzUpperLimitDampingUnits=N/(m/s)  PzUpperLimitTransitionRegionWidth=1e-4  PzUpperLimitTransitionRegionWidthUnits=m  PzPositionTargetSpecify=on  PzPositionTargetPriority=High  PzPositionTargetValue=xme_0(3)  PzPositionTargetValueUnits=m  PzVelocityTargetSpecify=on  PzVelocityTargetPriority=High  PzVelocityTargetValue=xme_dot_0(3)  PzVelocityTargetValueUnits=m/s  SphDefPosRotationMethod=None  SphDefPosRotationAngleUnits=deg  SphDefPosRotationStandardAxis=+Z  SphDefPosRotationAngle=0.0  SphDefPosRotationArbitraryAxis=[0 0 1]  SphDefPosFollAlignAxisA=+X  SphDefPosBaseAlignAxisA=+Y  SphDefPosFollAlignAxisB=+Y  SphDefPosBaseAlignAxisB=+Z  SphDefPosRotationSequenceAxes=FollowerAxes  SphDefPosRotationSequence=XYX  SphDefPosRotationSequenceAngles=[0 0 0]  SphDefPosRotationSequenceAnglesUnits=deg  SphDefPosRotationMatrix=[1 0 0; 0 1 0; 0 0 1]  SphEqPosRotationMethod=None  SphEqPosRotationAngleUnits=deg  SphEqPosRotationStandardAxis=+Z  SphEqPosRotationAngle=0.0  SphEqPosRotationArbitraryAxis=[0 0 1]  SphEqPosFollAlignAxisA=+X  SphEqPosBaseAlignAxisA=+Y  SphEqPosFollAlignAxisB=+Y  SphEqPosBaseAlignAxisB=+Z  SphEqPosRotationSequenceAxes=FollowerAxes  SphEqPosRotationSequence=XYX  SphEqPosRotationSequenceAngles=[0 0 0]  SphEqPosRotationSequenceAnglesUnits=deg  SphEqPosRotationMatrix=[1 0 0; 0 1 0; 0 0 1]  SphSpringStiffness=0  SphSpringStiffnessUnits=N*m/deg  SphDampingCoefficient=0  SphDampingCoefficientUnits=N*m/(deg/s)  SphActuateTorqueX=off  SphActuateTorqueY=off  SphActuateTorqueZ=off  SphActuateTorque=off  SphTorqueActuationMode=NoTorque  SphMotionActuationMode=ComputedMotion  SphActuationFrame=BaseFrame  SphSensePosition=off  SphSenseVelocityX=off  SphSenseVelocityY=off  SphSenseVelocityZ=off  SphSenseVelocity=off  SphSenseAccelerationX=off  SphSenseAccelerationY=off  SphSenseAccelerationZ=off  SphSenseAcceleration=off  SphSenseTorqueX=off  SphSenseTorqueY=off  SphSenseTorqueZ=off  SphSenseTorqueForce=off  SphSenseLowerLimitTorqueMag=off  SphSenseUpperLimitTorqueMag=off  SphSensingFrame=BaseFrame  SphLowerLimitSpecify=off  SphLowerLimitBound=15  SphLowerLimitBoundUnits=deg  SphLowerLimitStiffness=1e4  SphLowerLimitStiffnessUnits=N*m/deg  SphLowerLimitDamping=10  SphLowerLimitDampingUnits=N*m/(deg/s)  SphLowerLimitTransitionRegionWidth=0.1  SphLowerLimitTransitionRegionWidthUnits=deg  SphUpperLimitSpecify=off  SphUpperLimitBound=45  SphUpperLimitBoundUnits=deg  SphUpperLimitStiffness=1e4  SphUpperLimitStiffnessUnits=N*m/deg  SphUpperLimitDamping=10  SphUpperLimitDampingUnits=N*m/(deg/s)  SphUpperLimitTransitionRegionWidth=0.1  SphUpperLimitTransitionRegionWidthUnits=deg  SphPositionTargetRotationMethod=RotationSequence  SphPositionTargetRotationAngleUnits=deg  SphPositionTargetRotationStandardAxis=+Z  SphPositionTargetRotationAngle=0.0  SphPositionTargetRotationArbitraryAxis=[0 0 1]  SphPositionTargetFollAlignAxisA=+X  SphPositionTargetBaseAlignAxisA=+Y  SphPositionTargetFollAlignAxisB=+Y  SphPositionTargetBaseAlignAxisB=+Z  SphPositionTargetRotationSequenceAxes=FollowerAxes  SphPositionTargetRotationSequence=ZYX  SphPositionTargetRotationSequenceAngles=eul_0  SphPositionTargetRotationSequenceAnglesUnits=rad  SphPositionTargetRotationMatrix=[1 0 0; 0 1 0; 0 0 1]  SphPositionTargetSpecify=on  SphPositionTargetPriority=High  SphVelocityTargetValue=eul_dot_0  SphVelocityTargetValueUnits=rad/s  SphVelocityTargetSpecify=on  SphVelocityTargetPriority=High  SphVelocityTargetInFollowerFrame=on
      settings: AttributesFormatString=|
      | %<PxPositionTargetValue> %<PyPositionTargetValue> %<PzPositionTargetValue>
      | %<PxVelocityTargetValue> %<PyVelocityTargetValue> %<PzVelocityTargetValue>
      | %<SphPositionTargetRotationSequenceAngles>
      | %<SphPositionTargetRotationSequence>
      | %<SphVelocityTargetValue>
  Angular_MEAS : Subsystem
  Mux : Mux  Inputs=6
  PS-Simulink Converter : nesl_utility/PS-Simulink Converter  PhysicalDomain=network_engine_domain  SubClassName=ps_output  LeftPortType=input  RightPortType=output  PseudoPeriodic=off  Frequencies=[]  Unit=m  AffineConversion=off
      settings: SourceProductBaseCode=PW,SS
  PS-Simulink Converter1 : nesl_utility/PS-Simulink Converter  PhysicalDomain=network_engine_domain  SubClassName=ps_output  LeftPortType=input  RightPortType=output  PseudoPeriodic=off  Frequencies=[]  Unit=m  AffineConversion=off
      settings: SourceProductBaseCode=PW,SS
  PS-Simulink Converter2 : nesl_utility/PS-Simulink Converter  PhysicalDomain=network_engine_domain  SubClassName=ps_output  LeftPortType=input  RightPortType=output  PseudoPeriodic=off  Frequencies=[]  Unit=m  AffineConversion=off
      settings: SourceProductBaseCode=PW,SS
  PS-Simulink Converter3 : nesl_utility/PS-Simulink Converter  PhysicalDomain=network_engine_domain  SubClassName=ps_output  LeftPortType=input  RightPortType=output  PseudoPeriodic=off  Frequencies=[]  Unit=m/s  AffineConversion=off
      settings: SourceProductBaseCode=PW,SS
  PS-Simulink Converter4 : nesl_utility/PS-Simulink Converter  PhysicalDomain=network_engine_domain  SubClassName=ps_output  LeftPortType=input  RightPortType=output  PseudoPeriodic=off  Frequencies=[]  Unit=m/s  AffineConversion=off
      settings: SourceProductBaseCode=PW,SS
  PS-Simulink Converter5 : nesl_utility/PS-Simulink Converter  PhysicalDomain=network_engine_domain  SubClassName=ps_output  LeftPortType=input  RightPortType=output  PseudoPeriodic=off  Frequencies=[]  Unit=m/s  AffineConversion=off
      settings: SourceProductBaseCode=PW,SS
  Reshape : Reshape  OutputDimensionality=Column vector (2-D)
  Reshape1 : Reshape  OutputDimensionality=Column vector (2-D)
  Selector : Selector  InputPortWidth=6  IndexOptions=Index vector (dialog)  Indices=[1 3 5]  OutputSizes=1
  Selector1 : Selector  InputPortWidth=6  IndexOptions=Index vector (dialog)  Indices=[2 4 6]  OutputSizes=1
  integrate : Subsystem  Commented=on
  WORLD : PMIOPort  Side=Left
  AIRFRAME : PMIOPort  Port=2  Side=Right
  wb : Outport  VectorParamsAs1DForOutWhenUnconnected=off
  bRg : Outport  Port=2  VectorParamsAs1DForOutWhenUnconnected=off
  eul : Outport  Port=3  VectorParamsAs1DForOutWhenUnconnected=off
  eul_rates : Outport  Port=4  VectorParamsAs1DForOutWhenUnconnected=off
  Xe : Outport  Port=5  VectorParamsAs1DForOutWhenUnconnected=off
  Ve : Outport  Port=6  VectorParamsAs1DForOutWhenUnconnected=off
  wires:
  PS-Simulink Converter/1 -> Mux/1
  PS-Simulink Converter3/1 -> Mux/2
  PS-Simulink Converter1/1 -> Mux/3
  PS-Simulink Converter4/1 -> Mux/4
  PS-Simulink Converter2/1 -> Mux/5
  PS-Simulink Converter5/1 -> Mux/6
  Mux/1 -> Selector1/1, Selector/1
  Selector1/1 -> Reshape/1
  Selector/1 -> Reshape1/1
  Reshape1/1 -> Xe/1
  Reshape/1 -> Ve/1
  Angular_MEAS/1(wb) -> wb/1
  Angular_MEAS/2(bRg) -> bRg/1
  Angular_MEAS/3(eul) -> eul/1
  Angular_MEAS/4(eul_rates) -> eul_rates/1
  connections:
  PS-Simulink Converter4/LConn1 -- 6-DOF Joint/RConn5
  PS-Simulink Converter2/LConn1 -- 6-DOF Joint/RConn6
  PS-Simulink Converter/LConn1 -- 6-DOF Joint/RConn2
  PS-Simulink Converter3/LConn1 -- 6-DOF Joint/RConn3
  6-DOF Joint/LConn1 -- Angular_MEAS/LConn1 -- WORLD/RConn1
  PS-Simulink Converter5/LConn1 -- 6-DOF Joint/RConn7
  PS-Simulink Converter1/LConn1 -- 6-DOF Joint/RConn4
  6-DOF Joint/RConn1 -- Angular_MEAS/RConn1 -- AIRFRAME/RConn1

== system bh_compare_SM_vs_HAND_quad_and_spin_props/MODEL_SYS/bh_6DOF (Simscape)/Propellers ==
  note: ATTENTION:
      | The subsystems for propellers 1 and 3 are the same.
      | The subsystems for propellers 2 and 4 are the same
  mot_speed_vec : Inport
  Bus Creator : BusCreator  Inputs=4
  MOT_AERO_PROP_1 : Subsystem
      mask Display: image('wmot_pos.jpeg','center');
  MOT_AERO_PROP_2 : Subsystem
      mask Display: image('wmot_neg.jpeg','center');
  MOT_AERO_PROP_3 : Subsystem
      mask Display: image('wmot_pos.jpeg','center');
  MOT_AERO_PROP_4 : Subsystem
      mask Display: image('wmot_neg.jpeg','center');
  PROP_1 : sm_lib/Body Elements/Cylindrical Solid  GraphicAmbientColor=[0.15 0.15 0.15 1.0]  BasedOnType=Density  CenterOfMass=[0 0 0]  CenterOfMassUnits=m  GraphicDiffuseColor=[0.0 0.0 1.0]  CylinderLength=2*prop_CG_H  CylinderLengthUnits=m  CylinderRadius=prop_CG_H  CylinderRadiusUnits=m  Density=1000  DensityUnits=kg/(m^3)  DoExposeReferenceFrame=on  GraphicEmissiveColor=[0.0 0.0 0.0 1.0]  ExportEntireGeometry=off  SerializedFrames=<Frames/>  MarkerShape=Sphere  MarkerSize=10  GraphicType=FromGeometry  InertiaType=Custom  Mass=prop_mass  MassUnits=kg  MomentsOfInertia=Iprop_xx_yy_zz  MomentsOfInertiaUnits=kg*m^2  GraphicOpacity=1.0  ProductsOfInertia=Iprop_yz_zx_xy  ProductsOfInertiaUnits=kg*m^2  GraphicShininess=75  GraphicSpecularColor=[0.5 0.5 0.5 1.0]  GraphicVisPropType=SimpleVisualProperties
      settings: AttributesFormatString=|
      | %<Mass>
      | %<MomentsOfInertia>
      | %<ProductsOfInertia>
  PROP_2 : sm_lib/Body Elements/Cylindrical Solid  GraphicAmbientColor=[0.15 0.15 0.15 1.0]  BasedOnType=Density  CenterOfMass=[0 0 0]  CenterOfMassUnits=m  GraphicDiffuseColor=[0.8 0.8 1.0]  CylinderLength=2*prop_CG_H  CylinderLengthUnits=m  CylinderRadius=prop_CG_H  CylinderRadiusUnits=m  Density=1000  DensityUnits=kg/(m^3)  DoExposeReferenceFrame=on  GraphicEmissiveColor=[0.0 0.0 0.0 1.0]  ExportEntireGeometry=off  SerializedFrames=<Frames/>  MarkerShape=Sphere  MarkerSize=10  GraphicType=FromGeometry  InertiaType=Custom  Mass=prop_mass  MassUnits=kg  MomentsOfInertia=Iprop_xx_yy_zz  MomentsOfInertiaUnits=kg*m^2  GraphicOpacity=1.0  ProductsOfInertia=Iprop_yz_zx_xy  ProductsOfInertiaUnits=kg*m^2  GraphicShininess=75  GraphicSpecularColor=[0.5 0.5 0.5 1.0]  GraphicVisPropType=SimpleVisualProperties
      settings: AttributesFormatString=|
      | %<Mass>
      | %<MomentsOfInertia>
      | %<ProductsOfInertia>
  PROP_3 : sm_lib/Body Elements/Cylindrical Solid  GraphicAmbientColor=[0.15 0.15 0.15 1.0]  BasedOnType=Density  CenterOfMass=[0 0 0]  CenterOfMassUnits=m  GraphicDiffuseColor=[1.0 1.0 0.0]  CylinderLength=2*prop_CG_H  CylinderLengthUnits=m  CylinderRadius=prop_CG_H  CylinderRadiusUnits=m  Density=1000  DensityUnits=kg/(m^3)  DoExposeReferenceFrame=on  GraphicEmissiveColor=[0.0 0.0 0.0 1.0]  ExportEntireGeometry=off  SerializedFrames=<Frames/>  MarkerShape=Sphere  MarkerSize=10  GraphicType=FromGeometry  InertiaType=Custom  Mass=prop_mass  MassUnits=kg  MomentsOfInertia=Iprop_xx_yy_zz  MomentsOfInertiaUnits=kg*m^2  GraphicOpacity=1.0  ProductsOfInertia=Iprop_yz_zx_xy  ProductsOfInertiaUnits=kg*m^2  GraphicShininess=75  GraphicSpecularColor=[0.5 0.5 0.5 1.0]  GraphicVisPropType=SimpleVisualProperties
      settings: AttributesFormatString=|
      | %<Mass>
      | %<MomentsOfInertia>
      | %<ProductsOfInertia>
  PROP_4 : sm_lib/Body Elements/Cylindrical Solid  GraphicAmbientColor=[0.15 0.15 0.15 1.0]  BasedOnType=Density  CenterOfMass=[0 0 0]  CenterOfMassUnits=m  GraphicDiffuseColor=[0.2 1.0 1.0]  CylinderLength=2*prop_CG_H  CylinderLengthUnits=m  CylinderRadius=prop_CG_H  CylinderRadiusUnits=m  Density=1000  DensityUnits=kg/(m^3)  DoExposeReferenceFrame=on  GraphicEmissiveColor=[0.0 0.0 0.0 1.0]  ExportEntireGeometry=off  SerializedFrames=<Frames/>  MarkerShape=Sphere  MarkerSize=10  GraphicType=FromGeometry  InertiaType=Custom  Mass=prop_mass  MassUnits=kg  MomentsOfInertia=Iprop_xx_yy_zz  MomentsOfInertiaUnits=kg*m^2  GraphicOpacity=1.0  ProductsOfInertia=Iprop_yz_zx_xy  ProductsOfInertiaUnits=kg*m^2  GraphicShininess=75  GraphicSpecularColor=[0.5 0.5 0.5 1.0]  GraphicVisPropType=SimpleVisualProperties
      settings: AttributesFormatString=|
      | %<Mass>
      | %<MomentsOfInertia>
      | %<ProductsOfInertia>
  RT_air2prop1 : sm_lib/Frames and Transforms/Rigid Transform  TranslationMethod=Cartesian  TranslationStandardOffset=0  TranslationLengthUnit=m  TranslationStandardAxis=+Z  TranslationCartesianOffset=[prop_CG_L, 0, prop_CG_H]  TranslationROffset=0  TranslationROffsetUnits=m  TranslationZOffset=0  TranslationZOffsetUnits=m  TranslationThetaOffset=0  TranslationThetaOffsetUnits=deg  RotationMethod=None  RotationAngleUnits=deg  RotationStandardAxis=+Z  RotationAngle=0  RotationArbitraryAxis=[0 0 1]  FollAlignAxisA=+X  BaseAlignAxisA=+Y  FollAlignAxisB=+Y  BaseAlignAxisB=+Z  RotationSequenceAxes=FollowerAxes  RotationSequence=XYX  RotationSequenceAngles=[0 0 0]  RotationSequenceAnglesUnits=deg  RotationMatrix=[1 0 0; 0 1 0; 0 0 1]
  RT_air2prop2 : sm_lib/Frames and Transforms/Rigid Transform  TranslationMethod=Cartesian  TranslationStandardOffset=0  TranslationLengthUnit=m  TranslationStandardAxis=+Z  TranslationCartesianOffset=[0,prop_CG_L, prop_CG_H]  TranslationROffset=0  TranslationROffsetUnits=m  TranslationZOffset=0  TranslationZOffsetUnits=m  TranslationThetaOffset=0  TranslationThetaOffsetUnits=deg  RotationMethod=None  RotationAngleUnits=deg  RotationStandardAxis=+Z  RotationAngle=0  RotationArbitraryAxis=[0 0 1]  FollAlignAxisA=+X  BaseAlignAxisA=+Y  FollAlignAxisB=+Y  BaseAlignAxisB=+Z  RotationSequenceAxes=FollowerAxes  RotationSequence=XYX  RotationSequenceAngles=[0 0 0]  RotationSequenceAnglesUnits=deg  RotationMatrix=[1 0 0; 0 1 0; 0 0 1]
  RT_air2prop3 : sm_lib/Frames and Transforms/Rigid Transform  TranslationMethod=Cartesian  TranslationStandardOffset=0  TranslationLengthUnit=m  TranslationStandardAxis=+Z  TranslationCartesianOffset=[-prop_CG_L, 0, prop_CG_H]  TranslationROffset=0  TranslationROffsetUnits=m  TranslationZOffset=0  TranslationZOffsetUnits=m  TranslationThetaOffset=0  TranslationThetaOffsetUnits=deg  RotationMethod=None  RotationAngleUnits=deg  RotationStandardAxis=+Z  RotationAngle=0  RotationArbitraryAxis=[0 0 1]  FollAlignAxisA=+X  BaseAlignAxisA=+Y  FollAlignAxisB=+Y  BaseAlignAxisB=+Z  RotationSequenceAxes=FollowerAxes  RotationSequence=XYX  RotationSequenceAngles=[0 0 0]  RotationSequenceAnglesUnits=deg  RotationMatrix=[1 0 0; 0 1 0; 0 0 1]
  RT_air2prop4 : sm_lib/Frames and Transforms/Rigid Transform  TranslationMethod=Cartesian  TranslationStandardOffset=0  TranslationLengthUnit=m  TranslationStandardAxis=+Z  TranslationCartesianOffset=[0,-prop_CG_L, prop_CG_H]  TranslationROffset=0  TranslationROffsetUnits=m  TranslationZOffset=0  TranslationZOffsetUnits=m  TranslationThetaOffset=0  TranslationThetaOffsetUnits=deg  RotationMethod=None  RotationAngleUnits=deg  RotationStandardAxis=+Z  RotationAngle=0  RotationArbitraryAxis=[0 0 1]  FollAlignAxisA=+X  BaseAlignAxisA=+Y  FollAlignAxisB=+Y  BaseAlignAxisB=+Z  RotationSequenceAxes=FollowerAxes  RotationSequence=XYX  RotationSequenceAngles=[0 0 0]  RotationSequenceAnglesUnits=deg  RotationMatrix=[1 0 0; 0 1 0; 0 0 1]
  Selector4 : Selector  InputPortWidth=4  IndexOptions=Index vector (dialog)  Indices=1  OutputSizes=1
  Selector5 : Selector  InputPortWidth=4  IndexOptions=Index vector (dialog)  Indices=2  OutputSizes=1
  Selector6 : Selector  InputPortWidth=4  IndexOptions=Index vector (dialog)  Indices=3  OutputSizes=1
  Selector7 : Selector  InputPortWidth=4  IndexOptions=Index vector (dialog)  Indices=4  OutputSizes=1
  airCG : PMIOPort  Side=Left
  Prop_BUS : Outport  VectorParamsAs1DForOutWhenUnconnected=off
  wires:
  mot_speed_vec/1 -> [w]
  [w] -> Selector4/1
  Selector4/1 -> MOT_AERO_PROP_1/1(w_CMD_signed)
  [w] -> Selector6/1
  [w] -> Selector5/1
  [w] -> Selector7/1
  Selector5/1 -> MOT_AERO_PROP_2/1(w_CMD_signed)
  Selector6/1 -> MOT_AERO_PROP_3/1(w_CMD_signed)
  Selector7/1 -> MOT_AERO_PROP_4/1(w_CMD_signed)
  MOT_AERO_PROP_4/1(prop_BUS) -> [p4_bus]
  MOT_AERO_PROP_3/1(prop_BUS) -> [p3_bus]
  MOT_AERO_PROP_2/1(prop_BUS) -> [p2_bus]
  MOT_AERO_PROP_1/1(prop_BUS) -> [p1_bus]
  [p1_bus] -> Bus Creator/1  "prop_1"
  [p2_bus] -> Bus Creator/2  "prop_2"
  [p3_bus] -> Bus Creator/3  "prop_3"
  [p4_bus] -> Bus Creator/4  "prop_4"
  Bus Creator/1 -> Prop_BUS/1
  connections:
  MOT_AERO_PROP_1/LConn1 -- RT_air2prop1/RConn1
  MOT_AERO_PROP_1/RConn1 -- PROP_1/RConn1
  MOT_AERO_PROP_2/LConn1 -- RT_air2prop2/RConn1
  MOT_AERO_PROP_3/LConn1 -- RT_air2prop3/RConn1
  MOT_AERO_PROP_4/LConn1 -- RT_air2prop4/RConn1
  MOT_AERO_PROP_4/RConn1 -- PROP_4/RConn1
  MOT_AERO_PROP_3/RConn1 -- PROP_3/RConn1
  MOT_AERO_PROP_2/RConn1 -- PROP_2/RConn1
  airCG/RConn1 -- RT_air2prop4/LConn1 -- RT_air2prop3/LConn1 -- RT_air2prop1/LConn1 -- RT_air2prop2/LConn1

== system bh_compare_SM_vs_HAND_quad_and_spin_props/MODEL_SYS/bh_6DOF (Simscape)/echo_MASK_params ==
  Constant : Constant  Value=air_mass_0  OutDataTypeStr=Inherit: Inherit via back propagation
  Constant1 : Constant  Value=air_inertia_0  OutDataTypeStr=Inherit: Inherit via back propagation
  Constant11 : Constant  Value=xme_0  OutDataTypeStr=Inherit: Inherit via back propagation
  Constant2 : Constant  Value=prop_Imat  OutDataTypeStr=Inherit: Inherit via back propagation
  Constant3 : Constant  Value=prop_CG_L  OutDataTypeStr=Inherit: Inherit via back propagation
  Constant4 : Constant  Value=prop_CG_H  OutDataTypeStr=Inherit: Inherit via back propagation
  Constant5 : Constant  Value=prop_mass  OutDataTypeStr=Inherit: Inherit via back propagation
  Constant6 : Constant  Value=g_const  OutDataTypeStr=Inherit: Inherit via back propagation
  Constant7 : Constant  Value=eul_0  OutDataTypeStr=Inherit: Inherit via back propagation
  Constant8 : Constant  Value=Vm_0  OutDataTypeStr=Inherit: Inherit via back propagation
  Constant9 : Constant  Value=pm_0  OutDataTypeStr=Inherit: Inherit via back propagation
  Display{,1..10} (11 alike) : Display
  Reshape{1..3,5} (4 alike) : Reshape  OutputDimensionality=Column vector (2-D)
  wires:
  Constant2/1 -> Display1/1
  Constant1/1 -> Display/1
  Constant4/1 -> Display2/1
  Constant6/1 -> Display4/1
  Constant/1 -> Display5/1
  Constant5/1 -> Display6/1
  Constant3/1 -> Display3/1
  Constant7/1 -> Reshape5/1
  Reshape5/1 -> Display7/1
  Reshape1/1 -> Display8/1
  Constant9/1 -> Reshape1/1
  Reshape2/1 -> Display9/1
  Constant8/1 -> Reshape2/1
  Reshape3/1 -> Display10/1
  Constant11/1 -> Reshape3/1

== system bh_compare_SM_vs_HAND_quad_and_spin_props/CONT_SYS W_MOT_CMDS/MOTOR_sys/MOTOR_1/prefilter ==
  note: Y = U *     wn^2/( s^2 + 2*p*wn*s + wn^2)
      | Y*( s^2 + 2*p*wn*s + wn^2) = U * wn^2
      |
      | y'' + y'*2*p*wn + y*wn^2 = U*wn^2
  U : Inport
  Gain : Gain  Gain=2*p*wn
  Gain1 : Gain  Gain=wn^2
  Gain2 : Gain  Gain=wn^2
  Integrator : Integrator
  Integrator1 : Integrator
  Sum : Sum  Inputs=|+--
  U_filt : Outport  VectorParamsAs1DForOutWhenUnconnected=off
  U_DOT : Outport  Port=2  VectorParamsAs1DForOutWhenUnconnected=off
  wires:
  Integrator/1 -> Integrator1/1, [Y_DOT], Gain/1  "y_dot"
  Sum/1 -> Integrator/1  "y_dot_dot"
  Integrator1/1 -> Gain1/1, U_filt/1  "y"
  U/1 -> Gain2/1
  Gain2/1 -> Sum/1
  Gain/1 -> Sum/3
  Gain1/1 -> Sum/2
  [Y_DOT] -> U_DOT/1
